simulink library "TYPEBP_MASTER_tmp"  (Simulink 8.6)
settings: Solver=ode45  StartTime=0.0  StopTime=10.0  RelTol=1e-3
undefined symbols (not defined in the file): TYPEC, TYPEC_MASTER
libraries: cdsEpicsOut x112, cdsFilt x79, cdsTP x59, cdsFiltCtrl x36, VIS_LIB x20, cdsEpicsIn x18, cdsMuxMatrix x14, STATE_BIO_MASTER x12, cdsEpicsBinIn x8, cdsFunctionCall x4, lockin x4, cdsEpicsStringIn x2
(part 3 of 13)

== system TYPEBP_MASTER_tmp/TYPEBPMASTER_TEST/TEST ==
  In1 : Inport
  In4 : Inport  Port=2
  In7 : Inport  Port=3
  In10 : Inport  Port=4
  CH1 : cdsFiltCtrl/IIR FM with control  Tag=cdsFiltCtrl  Description=|
      | cdsFiltCntrl is the standard IIR filter module (exactly the same as cdsFilt) but with added control data output 'Ctrl'. Filter module digital signal output appears on the first output, which is called 'Val'. 'Ctrl' output has a bit pattern encoding the state of filter's on/off switches (FM1 through FM10). The bit values are:
      |                                                                                                                                                                                                                                                                                                                                       
      | module 	hex	dec                                                                                                                                                                                                                                                                                                                       
      | -----------------------                                                                                                                                                                                                                                                                                                               
      | FM1	0x20                    32                                                                                                                                                                                                                                                                                                        
      | FM2	0x80                     128                                                                                                                                                                                                                                                                                                      
      | FM3	0x200                   512                                                                                                                                                                                                                                                                                                       
      | FM4	0x800                   2048                                                                                                                                                                                                                                                                                                      
      | FM5	0x2000                 8192                                                                                                                                                                                                                                                                                                       
      | FM6	0x8000                 32768                                                                                                                                                                                                                                                                                                      
      | FM7	0x20000                131072                                                                                                                                                                                                                                                                                                     
      | FM8	0x80000                 524288                                                                                                                                                                                                                                                                                                    
      | FM9	0x200000               2097152                                                                                                                                                                                                                                                                                                    
      | FM10	0x800000               8388608                                                                                                                                                                                                                                                                                                   
      |                                                                                                                                                                                                                                                                                                                                       
      | This bit data can be used to drive some other switches or it can be output using a binary I/O module.
      settings: AttributesFormatString=%<Tag>
  CH2 : cdsFiltCtrl/IIR FM with control  Tag=cdsFiltCtrl  Description=|
      | cdsFiltCntrl is the standard IIR filter module (exactly the same as cdsFilt) but with added control data output 'Ctrl'. Filter module digital signal output appears on the first output, which is called 'Val'. 'Ctrl' output has a bit pattern encoding the state of filter's on/off switches (FM1 through FM10). The bit values are:
      |                                                                                                                                                                                                                                                                                                                                       
      | module 	hex	dec                                                                                                                                                                                                                                                                                                                       
      | -----------------------                                                                                                                                                                                                                                                                                                               
      | FM1	0x20                    32                                                                                                                                                                                                                                                                                                        
      | FM2	0x80                     128                                                                                                                                                                                                                                                                                                      
      | FM3	0x200                   512                                                                                                                                                                                                                                                                                                       
      | FM4	0x800                   2048                                                                                                                                                                                                                                                                                                      
      | FM5	0x2000                 8192                                                                                                                                                                                                                                                                                                       
      | FM6	0x8000                 32768                                                                                                                                                                                                                                                                                                      
      | FM7	0x20000                131072                                                                                                                                                                                                                                                                                                     
      | FM8	0x80000                 524288                                                                                                                                                                                                                                                                                                    
      | FM9	0x200000               2097152                                                                                                                                                                                                                                                                                                    
      | FM10	0x800000               8388608                                                                                                                                                                                                                                                                                                   
      |                                                                                                                                                                                                                                                                                                                                       
      | This bit data can be used to drive some other switches or it can be output using a binary I/O module.
      settings: AttributesFormatString=%<Tag>
  CH3 : cdsFiltCtrl/IIR FM with control  Tag=cdsFiltCtrl  Description=|
      | cdsFiltCntrl is the standard IIR filter module (exactly the same as cdsFilt) but with added control data output 'Ctrl'. Filter module digital signal output appears on the first output, which is called 'Val'. 'Ctrl' output has a bit pattern encoding the state of filter's on/off switches (FM1 through FM10). The bit values are:
      |                                                                                                                                                                                                                                                                                                                                       
      | module 	hex	dec                                                                                                                                                                                                                                                                                                                       
      | -----------------------                                                                                                                                                                                                                                                                                                               
      | FM1	0x20                    32                                                                                                                                                                                                                                                                                                        
      | FM2	0x80                     128                                                                                                                                                                                                                                                                                                      
      | FM3	0x200                   512                                                                                                                                                                                                                                                                                                       
      | FM4	0x800                   2048                                                                                                                                                                                                                                                                                                      
      | FM5	0x2000                 8192                                                                                                                                                                                                                                                                                                       
      | FM6	0x8000                 32768                                                                                                                                                                                                                                                                                                      
      | FM7	0x20000                131072                                                                                                                                                                                                                                                                                                     
      | FM8	0x80000                 524288                                                                                                                                                                                                                                                                                                    
      | FM9	0x200000               2097152                                                                                                                                                                                                                                                                                                    
      | FM10	0x800000               8388608                                                                                                                                                                                                                                                                                                   
      |                                                                                                                                                                                                                                                                                                                                       
      | This bit data can be used to drive some other switches or it can be output using a binary I/O module.
      settings: AttributesFormatString=%<Tag>
  CH4 : cdsFiltCtrl/IIR FM with control  Tag=cdsFiltCtrl  Description=|
      | cdsFiltCntrl is the standard IIR filter module (exactly the same as cdsFilt) but with added control data output 'Ctrl'. Filter module digital signal output appears on the first output, which is called 'Val'. 'Ctrl' output has a bit pattern encoding the state of filter's on/off switches (FM1 through FM10). The bit values are:
      |                                                                                                                                                                                                                                                                                                                                       
      | module 	hex	dec                                                                                                                                                                                                                                                                                                                       
      | -----------------------                                                                                                                                                                                                                                                                                                               
      | FM1	0x20                    32                                                                                                                                                                                                                                                                                                        
      | FM2	0x80                     128                                                                                                                                                                                                                                                                                                      
      | FM3	0x200                   512                                                                                                                                                                                                                                                                                                       
      | FM4	0x800                   2048                                                                                                                                                                                                                                                                                                      
      | FM5	0x2000                 8192                                                                                                                                                                                                                                                                                                       
      | FM6	0x8000                 32768                                                                                                                                                                                                                                                                                                      
      | FM7	0x20000                131072                                                                                                                                                                                                                                                                                                     
      | FM8	0x80000                 524288                                                                                                                                                                                                                                                                                                    
      | FM9	0x200000               2097152                                                                                                                                                                                                                                                                                                    
      | FM10	0x800000               8388608                                                                                                                                                                                                                                                                                                   
      |                                                                                                                                                                                                                                                                                                                                       
      | This bit data can be used to drive some other switches or it can be output using a binary I/O module.
      settings: AttributesFormatString=%<Tag>
  Ground{1..6,19,22} (8 alike) : Ground
  Terminator{1..5,16..18} (8 alike) : Terminator
  wires:
  CH4/2 -> Terminator1/1
  Ground5/1 -> CH4/3
  Ground6/1 -> CH4/2
  Ground3/1 -> CH3/3
  Ground4/1 -> CH3/2
  Ground1/1 -> CH2/3
  Ground2/1 -> CH2/2
  CH3/2 -> Terminator18/1
  CH2/2 -> Terminator17/1
  CH1/2 -> Terminator16/1
  Ground19/1 -> CH1/3
  Ground22/1 -> CH1/2
  In10/1 -> CH4/1
  In7/1 -> CH3/1
  In1/1 -> CH1/1
  CH2/1 -> Terminator4/1
  In4/1 -> CH2/1
  CH4/1 -> Terminator2/1
  CH3/1 -> Terminator3/1
  CH1/1 -> Terminator5/1

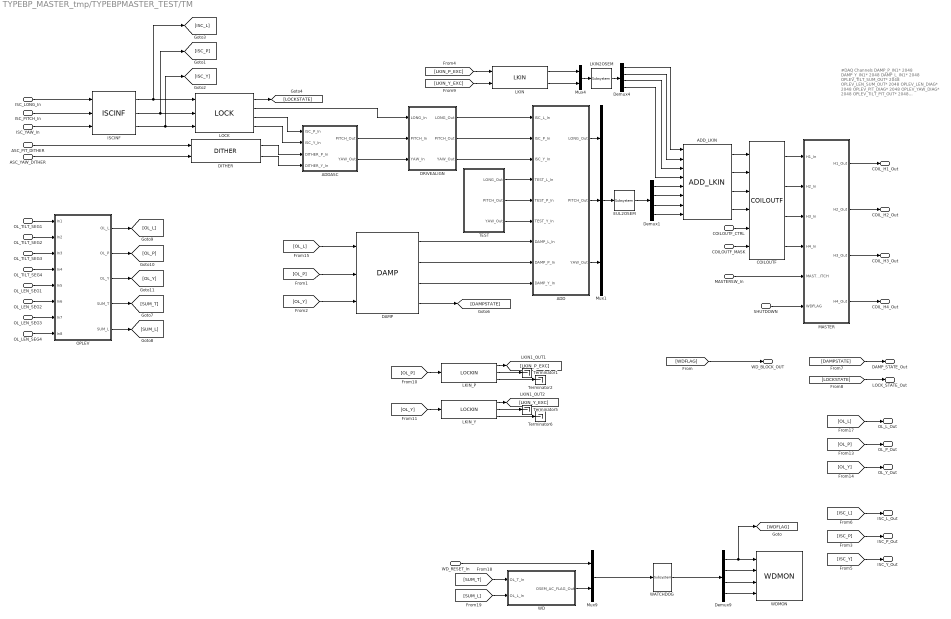
== system TYPEBP_MASTER_tmp/TYPEBPMASTER_TEST/TM ==
  note: #DAQ Channels
      | DAMP_P_IN1* 2048
      | DAMP_Y_IN1* 2048
      | DAMP_L_IN1* 2048
      | OPLEV_TILT_SUM_OUT* 2048
      | OPLEV_LEN_SUM_OUT* 2048
      | OPLEV_LEN_DIAG* 2048
      | OPLEV_PIT_DIAG* 2048
      | OPLEV_YAW_DIAG* 2048
      | OPLEV_TILT_PIT_OUT* 2048
      | OPLEV_TILT_YAW_OUT* 2048
      | ISCINF_L_IN1 2048
  ISC_LONG_In : Inport
  ISC_PITCH_In : Inport  Port=2
  ISC_YAW_In : Inport  Port=3
  COILOUTF_CTRL : Inport  Port=4
  COILOUTF_MASK : Inport  Port=5
  OL_TILT_SEG1 : Inport  Port=6
  OL_TILT_SEG2 : Inport  Port=7
  OL_TILT_SEG3 : Inport  Port=8
  OL_TILT_SEG4 : Inport  Port=9
  OL_LEN_SEG1 : Inport  Port=10
  OL_LEN_SEG2 : Inport  Port=11
  OL_LEN_SEG3 : Inport  Port=12
  OL_LEN_SEG4 : Inport  Port=13
  MASTERSW_In : Inport  Port=14
  WD_RESET_In : Inport  Port=15
  ASC_PIT_DITHER : Inport  Port=16
  ASC_YAW_DITHER : Inport  Port=17
  SHUTDOWN : Inport  Port=18
  ADD : Subsystem
  ADDASC : Subsystem
  ADD_LKIN : VIS_LIB/ADD_LKIN
  COILOUTF : FOUROSEM_COILOUTF_MASTER/COILOUTF
  DAMP : VIS_LIB/DAMP
  DITHER : VIS_LIB/DITHER
  DRIVEALIGN : Subsystem
  Demux1 : Demux
  Demux4 : Demux
  Demux9 : Demux
  EUL2OSEM : cdsMuxMatrix/Subsystem  Tag=cdsMuxMatrix  Description=Any size matrix. Inputs and outputs must be connected using Mux and Demux parts.
      settings: AttributesFormatString=%<Tag>
  ISCINF : VIS_LIB/ISCINF
  LKIN : VIS_LIB/LKIN
  LKIN2OSEM : cdsMuxMatrix/Subsystem  Tag=cdsMuxMatrix  Description=Any size matrix. Inputs and outputs must be connected using Mux and Demux parts.
      settings: AttributesFormatString=%<Tag>
  LKIN_P : lockin/LOCKIN  Description=ADL=LOCKIN.adl
      settings: AttributesFormatString=%<Tag>
  LKIN_Y : lockin/LOCKIN  Description=ADL=LOCKIN.adl
      settings: AttributesFormatString=%<Tag>
  LOCK : VIS_LIB/LOCK
  MASTER : Subsystem  AncestorBlock=CRYP_TM_MASTER/CRYP_TM_MASTER/MASTER
  Mux1 : Mux  Inputs=3
  Mux4 : Mux  Inputs=2
  Mux9 : Mux  Inputs=2
  OPLEV : Subsystem
  TEST : Subsystem
  Terminator{1..2,5..6} (4 alike) : Terminator
  WATCHDOG : cdsFunctionCall/Subsystem  Tag=cdsFunctionCall  Description=inline OSEMWATCHDOG /opt/rtcds/userapps/release/vis/common/src/WATCHDOG.c
      settings: AttributesFormatString=%<Tag>\n%<Description>
  WD : Subsystem
  WDMON : VIS_LIB/WDMON
  COIL_H1_Out : Outport
  COIL_H2_Out : Outport  Port=2
  COIL_H3_Out : Outport  Port=3
  COIL_H4_Out : Outport  Port=4
  WD_BLOCK_OUT : Outport  Port=5
  DAMP_STATE_Out : Outport  Port=6
  LOCK_STATE_Out : Outport  Port=7
  OL_L_Out : Outport  Port=8
  OL_P_Out : Outport  Port=9
  OL_Y_Out : Outport  Port=10
  ISC_L_Out : Outport  Port=11
  ISC_P_Out : Outport  Port=12
  ISC_Y_Out : Outport  Port=13
  wires:
  [ISC_L] -> ISC_L_Out/1
  [ISC_P] -> ISC_P_Out/1
  [ISC_Y] -> ISC_Y_Out/1
  ISCINF/3 -> LOCK/3, [ISC_Y]
  ISCINF/2 -> LOCK/2, [ISC_P]
  ISCINF/1 -> LOCK/1, [ISC_L]
  [OL_Y] -> DAMP/3
  [OL_P] -> DAMP/2
  DAMP/3 -> ADD/9(DAMP_Y_In)
  DAMP/2 -> ADD/8(DAMP_P_In)
  OPLEV/3(OL_Y) -> [OL_Y]
  OPLEV/2(OL_P) -> [OL_P]
  OPLEV/1(OL_L) -> [OL_L]
  [OL_L] -> OL_L_Out/1
  [SUM_L] -> WD/2(OL_L_In)
  OPLEV/5(SUM_L) -> [SUM_L]
  OPLEV/4(SUM_T) -> [SUM_T]
  [SUM_T] -> WD/1(OL_T_In)
  DAMP/1 -> ADD/7(DAMP_L_In)
  DAMP/4 -> [DAMPSTATE]
  [OL_L] -> DAMP/1
  OL_TILT_SEG3/1 -> OPLEV/3(In3)
  OL_LEN_SEG4/1 -> OPLEV/8(In8)
  OL_LEN_SEG3/1 -> OPLEV/7(In7)
  OL_LEN_SEG2/1 -> OPLEV/6(In6)
  OL_LEN_SEG1/1 -> OPLEV/5(In5)
  OL_TILT_SEG4/1 -> OPLEV/4(In4)
  OL_TILT_SEG2/1 -> OPLEV/2(In2)
  OL_TILT_SEG1/1 -> OPLEV/1(In1)
  LOCK/3 -> ADDASC/1(ISC_P_In)
  TEST/3(YAW_Out) -> ADD/6(TEST_Y_In)
  TEST/2(PITCH_Out) -> ADD/5(TEST_P_In)
  TEST/1(LONG_Out) -> ADD/4(TEST_L_In)
  COILOUTF_CTRL/1 -> COILOUTF/5
  COILOUTF_MASK/1 -> COILOUTF/6
  WD_RESET_In/1 -> Mux9/1
  COILOUTF/4 -> MASTER/4(H4_In)
  COILOUTF/3 -> MASTER/3(H3_In)
  COILOUTF/2 -> MASTER/2(H2_In)
  COILOUTF/1 -> MASTER/1(H1_In)
  [WDFLAG] -> WD_BLOCK_OUT/1
  Mux9/1 -> WATCHDOG/1
  WATCHDOG/1 -> Demux9/1
  Demux9/4 -> WDMON/4
  Demux9/3 -> WDMON/3
  Demux9/2 -> WDMON/2
  Demux9/1 -> WDMON/1, [WDFLAG]
  EUL2OSEM/1 -> Demux1/1
  Mux1/1 -> EUL2OSEM/1
  ASC_PIT_DITHER/1 -> DITHER/1
  ASC_YAW_DITHER/1 -> DITHER/2
  LOCK/4 -> ADDASC/2(ISC_Y_In)
  DITHER/1 -> ADDASC/3(DITHER_P_In)
  DITHER/2 -> ADDASC/4(DITHER_Y_In)
  ADD/3(YAW_Out) -> Mux1/3
  ADD/2(PITCH_Out) -> Mux1/2
  ADD/1(LONG_Out) -> Mux1/1
  LOCK/2 -> DRIVEALIGN/1(LONG_In)
  ADDASC/1(PITCH_Out) -> DRIVEALIGN/2(PITCH_In)
  ADDASC/2(YAW_Out) -> DRIVEALIGN/3(YAW_In)
  DRIVEALIGN/1(LONG_Out) -> ADD/1(ISC_L_In)
  DRIVEALIGN/2(PITCH_Out) -> ADD/2(ISC_P_In)
  DRIVEALIGN/3(YAW_Out) -> ADD/3(ISC_Y_In)
  MASTER/1(H1_Out) -> COIL_H1_Out/1
  MASTER/2(H2_Out) -> COIL_H2_Out/1
  MASTER/3(H3_Out) -> COIL_H3_Out/1
  MASTER/4(H4_Out) -> COIL_H4_Out/1
  Mux4/1 -> LKIN2OSEM/1
  LKIN2OSEM/1 -> Demux4/1
  Demux4/1 -> ADD_LKIN/1
  LKIN/1 -> Mux4/1
  LKIN/2 -> Mux4/2
  Demux4/2 -> ADD_LKIN/2
  Demux4/3 -> ADD_LKIN/3
  Demux4/4 -> ADD_LKIN/4
  Demux1/1 -> ADD_LKIN/5
  Demux1/2 -> ADD_LKIN/6
  Demux1/3 -> ADD_LKIN/7
  Demux1/4 -> ADD_LKIN/8
  ADD_LKIN/1 -> COILOUTF/1
  ADD_LKIN/2 -> COILOUTF/2
  ADD_LKIN/3 -> COILOUTF/3
  ADD_LKIN/4 -> COILOUTF/4
  MASTERSW_In/1 -> MASTER/5(MASTERSWITCH)
  [DAMPSTATE] -> DAMP_STATE_Out/1
  [LOCKSTATE] -> LOCK_STATE_Out/1
  LOCK/1 -> [LOCKSTATE]
  [OL_P] -> LKIN_P/1
  LKIN_P/2 -> Terminator1/1
  LKIN_P/3 -> Terminator2/1
  LKIN_P/1 -> [LKIN_P_EXC]
  LKIN_Y/1 -> [LKIN_Y_EXC]
  [OL_Y] -> LKIN_Y/1
  LKIN_Y/2 -> Terminator5/1
  LKIN_Y/3 -> Terminator6/1
  [LKIN_P_EXC] -> LKIN/1
  [LKIN_Y_EXC] -> LKIN/2
  WD/1(OSEM_AC_FLAG_Out) -> Mux9/2
  ISC_YAW_In/1 -> ISCINF/3
  ISC_LONG_In/1 -> ISCINF/1
  ISC_PITCH_In/1 -> ISCINF/2
  [OL_P] -> OL_P_Out/1
  [OL_Y] -> OL_Y_Out/1
  SHUTDOWN/1 -> MASTER/6(WDFLAG)

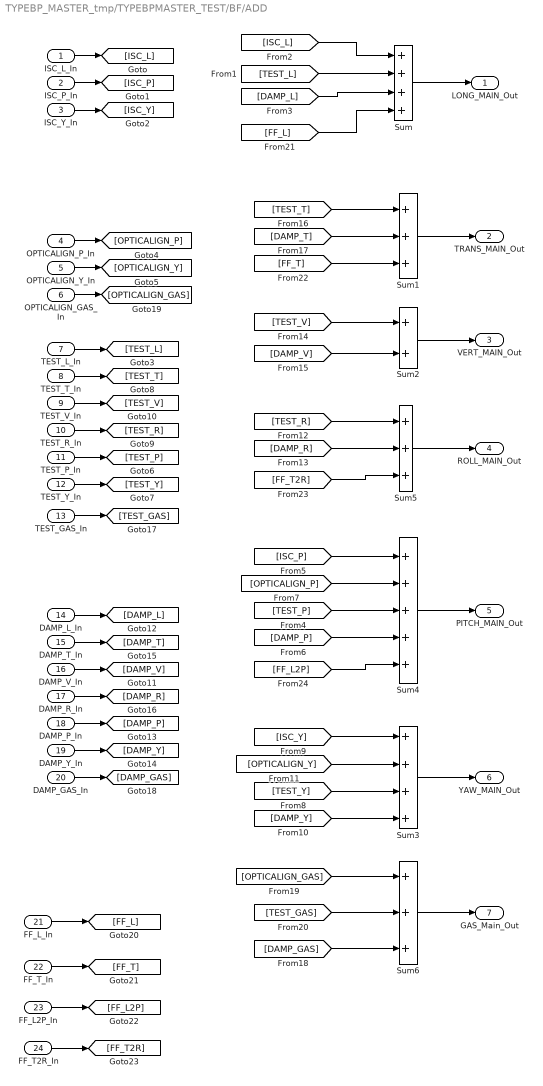
== system TYPEBP_MASTER_tmp/TYPEBPMASTER_TEST/BF/ADD ==
  ISC_L_In : Inport
  ISC_P_In : Inport  Port=2
  ISC_Y_In : Inport  Port=3
  OPTICALIGN_P_In : Inport  Port=4
  OPTICALIGN_Y_In : Inport  Port=5
  OPTICALIGN_GAS_In : Inport  Port=6
  TEST_L_In : Inport  Port=7
  TEST_T_In : Inport  Port=8
  TEST_V_In : Inport  Port=9
  TEST_R_In : Inport  Port=10
  TEST_P_In : Inport  Port=11
  TEST_Y_In : Inport  Port=12
  TEST_GAS_In : Inport  Port=13
  DAMP_L_In : Inport  Port=14
  DAMP_T_In : Inport  Port=15
  DAMP_V_In : Inport  Port=16
  DAMP_R_In : Inport  Port=17
  DAMP_P_In : Inport  Port=18
  DAMP_Y_In : Inport  Port=19
  DAMP_GAS_In : Inport  Port=20
  FF_L_In : Inport  Port=21
  FF_T_In : Inport  Port=22
  FF_L2P_In : Inport  Port=23
  FF_T2R_In : Inport  Port=24
  Sum : Sum  Inputs=++++
  Sum1 : Sum  Inputs=+++
  Sum2 : Sum
  Sum3 : Sum  Inputs=++++
  Sum4 : Sum  Inputs=+++++
  Sum5 : Sum  Inputs=+++
  Sum6 : Sum  Inputs=+++
  LONG_MAIN_Out : Outport
  TRANS_MAIN_Out : Outport  Port=2
  VERT_MAIN_Out : Outport  Port=3
  ROLL_MAIN_Out : Outport  Port=4
  PITCH_MAIN_Out : Outport  Port=5
  YAW_MAIN_Out : Outport  Port=6
  GAS_Main_Out : Outport  Port=7
  wires:
  FF_T2R_In/1 -> [FF_T2R]
  [FF_L2P] -> Sum4/5
  [FF_T2R] -> Sum5/3
  FF_L2P_In/1 -> [FF_L2P]
  [FF_T] -> Sum1/3
  [FF_L] -> Sum/4
  FF_T_In/1 -> [FF_T]
  FF_L_In/1 -> [FF_L]
  [DAMP_GAS] -> Sum6/3
  [TEST_GAS] -> Sum6/2
  [OPTICALIGN_GAS] -> Sum6/1
  DAMP_GAS_In/1 -> [DAMP_GAS]
  DAMP_Y_In/1 -> [DAMP_Y]
  DAMP_P_In/1 -> [DAMP_P]
  DAMP_R_In/1 -> [DAMP_R]
  DAMP_V_In/1 -> [DAMP_V]
  DAMP_T_In/1 -> [DAMP_T]
  DAMP_L_In/1 -> [DAMP_L]
  TEST_GAS_In/1 -> [TEST_GAS]
  TEST_Y_In/1 -> [TEST_Y]
  TEST_P_In/1 -> [TEST_P]
  TEST_R_In/1 -> [TEST_R]
  TEST_V_In/1 -> [TEST_V]
  TEST_T_In/1 -> [TEST_T]
  TEST_L_In/1 -> [TEST_L]
  OPTICALIGN_GAS_In/1 -> [OPTICALIGN_GAS]
  Sum6/1 -> GAS_Main_Out/1
  Sum4/1 -> PITCH_MAIN_Out/1
  Sum3/1 -> YAW_MAIN_Out/1
  Sum/1 -> LONG_MAIN_Out/1
  [ISC_L] -> Sum/1
  [TEST_L] -> Sum/2
  [DAMP_L] -> Sum/3
  Sum5/1 -> ROLL_MAIN_Out/1
  Sum2/1 -> VERT_MAIN_Out/1
  Sum1/1 -> TRANS_MAIN_Out/1
  OPTICALIGN_P_In/1 -> [OPTICALIGN_P]
  OPTICALIGN_Y_In/1 -> [OPTICALIGN_Y]
  ISC_L_In/1 -> [ISC_L]
  ISC_P_In/1 -> [ISC_P]
  ISC_Y_In/1 -> [ISC_Y]
  [ISC_P] -> Sum4/1
  [OPTICALIGN_P] -> Sum4/2
  [TEST_P] -> Sum4/3
  [DAMP_P] -> Sum4/4
  [ISC_Y] -> Sum3/1
  [OPTICALIGN_Y] -> Sum3/2
  [TEST_Y] -> Sum3/3
  [DAMP_Y] -> Sum3/4
  [TEST_R] -> Sum5/1
  [DAMP_R] -> Sum5/2
  [TEST_T] -> Sum1/1
  [DAMP_T] -> Sum1/2
  [TEST_V] -> Sum2/1
  [DAMP_V] -> Sum2/2
